simulink model "HEV"  (R2015a)
settings: Solver=ode23tb  StartTime=0.0  StopTime=318  FixedStep=Ts  MaxStep=Ts  RelTol=1  AbsTol=0.5
InitFcn:
  | Ts = 6e-05;   % time step
  | DriveCycleNumber = 1;
  | beginningSim = 1;
undefined symbols (not defined in the file): drive_block, drive_enginemodel, EngineSpeedPower, FuelConsTable, GasEmisTable, h, Hydride, km, magnitude, Metal, Nickel, rad, s, speed, torque
libraries: powerlib x47, driveline x30, simulink x13, simulink_extras x9, electricdrivelib x3, powerlib_extras x3, aerolibconvert2 x2, DC6DriveInternalModels x1
(part 3 of 3)

== system HEV/Electric Motor Controller /Motor 50kW/Three-phase Inverter/Activation Switches ==
  gate : Inport
  Ideal Switch1 : powerlib/Power Electronics/Ideal Switch  Ron=2*Ron  Lon=0  IC=1  Rs=1e6  Cs=inf  Measurements=off
  Ideal Switch2 : powerlib/Power Electronics/Ideal Switch  Ron=2*Ron  Lon=0  IC=1  Rs=1e6  Cs=inf  Measurements=off
  Ideal Switch3 : powerlib/Power Electronics/Ideal Switch  Ron=2*Ron  Lon=0  IC=1  Rs=1e6  Cs=inf  Measurements=off
  Ideal Switch4 : powerlib/Power Electronics/Ideal Switch  Ron=2*Ron  Lon=0  IC=0  Rs=1e6  Cs=inf  Measurements=off
  Ideal Switch5 : powerlib/Power Electronics/Ideal Switch  Ron=2*Ron  Lon=0  IC=0  Rs=1e6  Cs=inf  Measurements=off
  Ideal Switch6 : powerlib/Power Electronics/Ideal Switch  Ron=2*Ron  Lon=0  IC=0  Rs=1e6  Cs=inf  Measurements=off
  Logical Operator : Logic  Operator=NOT  AllPortsSameDT=off  OutDataTypeStr=boolean
  A1 : PMIOPort  Port=1  Side=Left
  a : PMIOPort  Port=2  Side=Right
  B1 : PMIOPort  Port=3  Side=Left
  b : PMIOPort  Port=4  Side=Right
  C1 : PMIOPort  Port=5  Side=Left
  c : PMIOPort  Port=6  Side=Right
  A2 : PMIOPort  Port=7  Side=Left
  B2 : PMIOPort  Port=8  Side=Left
  C2 : PMIOPort  Port=9  Side=Left
  wires:
  gate/1 -> Ideal Switch1/1, Ideal Switch2/1, Ideal Switch3/1, Logical Operator/1
  Logical Operator/1 -> Ideal Switch4/1, Ideal Switch5/1, Ideal Switch6/1
  connections:
  A1/RConn1 -- Ideal Switch1/LConn1
  Ideal Switch1/RConn1 -- a/RConn1 -- Ideal Switch4/RConn1
  B1/RConn1 -- Ideal Switch2/LConn1
  Ideal Switch2/RConn1 -- Ideal Switch5/RConn1 -- b/RConn1
  C1/RConn1 -- Ideal Switch3/LConn1
  Ideal Switch3/RConn1 -- Ideal Switch6/RConn1 -- c/RConn1
  A2/RConn1 -- Ideal Switch4/LConn1
  B2/RConn1 -- Ideal Switch5/LConn1
  C2/RConn1 -- Ideal Switch6/LConn1

== system HEV/Electric Motor Controller /Motor 50kW/Three-phase Inverter/Id computation ==
  m : Inport
  Vdc : Inport  Port=2
  Demux : Subsystem
  Demux1 : Subsystem
  Gain : Gain  Gain=Ron
  Math Function : Math  Operator=magnitude^2  SaturateOnIntegerOverflow=on
  Math Function1 : Math  Operator=magnitude^2  SaturateOnIntegerOverflow=on
  Math Function2 : Math  Operator=magnitude^2  SaturateOnIntegerOverflow=on
  Product1 : Product  Inputs=*/  SaturateOnIntegerOverflow=on  OutDataTypeStr=Inherit: Same as first input
  Sum1 : Sum  Inputs=+++  SaturateOnIntegerOverflow=on
  Sum2 : Sum  Inputs=|++  SaturateOnIntegerOverflow=on
  Sum3 : Sum  SaturateOnIntegerOverflow=on
  Unit Delay1 : UnitDelay  SampleTime=Ts
  Unit Delay4 : UnitDelay  InitialCondition=1  SampleTime=Ts
  Vac x Ia : Product  SaturateOnIntegerOverflow=on  OutDataTypeStr=Inherit: Same as first input
  Vbc x Ib : Product  SaturateOnIntegerOverflow=on  OutDataTypeStr=Inherit: Same as first input
  Zero avoider : Saturate  UpperLimit=inf  LowerLimit=1
  Id : Outport
  wires:
  Sum2/1 -> Unit Delay1/1
  Sum3/1 -> Sum2/1
  Sum1/1 -> Gain/1
  Math Function2/1 -> Sum1/3
  Math Function/1 -> Sum1/1
  Math Function1/1 -> Sum1/2
  Demux1/3(Ic) -> Math Function2/1
  Demux1/2(Ib) -> Math Function1/1
  Demux1/1(Ia) -> Math Function/1
  Unit Delay4/1 -> Zero avoider/1
  Unit Delay1/1 -> Product1/1
  m/1 -> Demux1/1(m), Demux/1(m)
  Vac x Ia/1 -> Sum3/1
  Vbc x Ib/1 -> Sum3/2
  Vdc/1 -> Unit Delay4/1
  Demux/1(Vac) -> Vac x Ia/1
  Demux/2(Ia) -> Vac x Ia/2
  Demux/4(Ib) -> Vbc x Ib/2
  Demux/3(Vbc) -> Vbc x Ib/1
  Gain/1 -> Sum2/2
  Product1/1 -> Id/1
  Zero avoider/1 -> Product1/2

== system HEV/Electric Motor Controller /Motor 50kW/Three-phase Inverter/Limit detection ==
  note: Limit = 1 saturation mode (voltage mode)
      | Limit = 0 normal mode (current mode)
  note: Low pass filter
  note: Low pass filter
  Vcc : Inport
  ctrl : Inport  Port=2
  Bus Selector1 : BusSelector  OutputSignals=m.Stator current is_d (A),m.Stator current is_q (A),m.Rotor speed wm (rad/s)  OutputAsBus=on
  Discrete Transfer Fcn1 : DiscreteTransferFcn  Numerator=[1-exp(-Ts*Fcs*2*pi)]  Denominator=[1 -exp(-Ts*Fcs*2*pi)]  SampleTime=Ts
  Discrete Transfer Fcn3 : DiscreteTransferFcn  Numerator=[1-exp(-Ts*Fcs*2*pi)]  Denominator=[1 -exp(-Ts*Fcs*2*pi)]  SampleTime=Ts
  Gain1 : Gain  Gain=0.9  SaturateOnIntegerOverflow=on  OutDataTypeStr=Inherit: Same as input  ParamDataTypeStr=Inherit: Same as input
  "Internal Vcc " : Fcn  Expr=pi/2*sqrt((Resistance*u(1)-Lq*p*u(3)*u(2))^2+(Resistance*u(2)+Ld*p*u(3)*u(1)+Flux*p*u(3))^2)
  Relational Operator : RelationalOperator  Operator=>  OutDataTypeStr=boolean
  Relational Operator2 : RelationalOperator  Operator=<  OutDataTypeStr=boolean
  S-R Flip-Flop : simulink_extras/Flip Flops/S-R Flip-Flop  initial_condition=0
  Terminator : Terminator
  Limit : Outport
  wires:
  Vcc/1 -> Discrete Transfer Fcn3/1
  Relational Operator/1 -> S-R Flip-Flop/1
  Relational Operator2/1 -> S-R Flip-Flop/2
  S-R Flip-Flop/1 -> Limit/1
  ctrl/1 -> Bus Selector1/1
  Bus Selector1/1 -> "Internal Vcc "/1
  "Internal Vcc "/1 -> Discrete Transfer Fcn1/1
  Discrete Transfer Fcn1/1 -> Relational Operator/1, Relational Operator2/1
  Gain1/1 -> Relational Operator2/2
  Discrete Transfer Fcn3/1 -> Gain1/1, Relational Operator/2
  S-R Flip-Flop/2 -> Terminator/1

== system HEV/Electric Motor Controller /Motor 50kW/Three-phase Inverter/Output Resistance correction ==
  note: Vabc
  ctrl : Inport
  1/R : Gain  Gain=1/(100*Resistance)  SaturateOnIntegerOverflow=on  OutDataTypeStr=Inherit: Same as input  ParamDataTypeStr=Inherit: Same as input
  Bus Selector1 : BusSelector  OutputSignals=m.Stator voltage Vs_d (V),m.Stator voltage Vs_q (V),m.Rotor angle thetam (rad)
  Constant : Constant  Value=0
  Discrete Transfer Fcn1 : DiscreteTransferFcn  Numerator=[1-exp(-Ts/.001)]  Denominator=[1 -exp(-Ts/.001)]  SampleTime=Ts
  Discrete Transfer Fcn2 : DiscreteTransferFcn  Numerator=[1-exp(-Ts/.001)]  Denominator=[1 -exp(-Ts/.001)]  SampleTime=Ts
  Fcn : Fcn  Expr=sin(u)
  Fcn1 : Fcn  Expr=cos(u)
  Mux4 : Mux  Inputs=3
  Mux5 : Mux  Inputs=2
  dq0_to_abc Transformation : powerlib_extras/Measurements/dq0_to_abc Transformation
  poles : Gain  Gain=p  SaturateOnIntegerOverflow=on  OutDataTypeStr=Inherit: Same as input  ParamDataTypeStr=Inherit: Same as input
  "Iabc_r " : Outport
  wires:
  1/R/1 -> "Iabc_r "/1
  Bus Selector1/2 -> Discrete Transfer Fcn2/1  "<Stator voltage Vs_q (V)>"
  Bus Selector1/1 -> Discrete Transfer Fcn1/1  "<Stator voltage Vs_d (V)>"
  ctrl/1 -> Bus Selector1/1
  Mux4/1 -> dq0_to_abc Transformation/1
  Fcn/1 -> Mux5/1
  Fcn1/1 -> Mux5/2
  Mux5/1 -> dq0_to_abc Transformation/2
  Constant/1 -> Mux4/3
  dq0_to_abc Transformation/1 -> 1/R/1
  Discrete Transfer Fcn2/1 -> Mux4/2
  Discrete Transfer Fcn1/1 -> Mux4/1
  Bus Selector1/3 -> poles/1  "<Rotor angle thetam (rad)>"
  poles/1 -> Fcn1/1, Fcn/1

== system HEV/Electric Motor Controller /Motor 50kW/VECT controller/Current Regulator ==
  Iabc* : Inport
  Iabc : Inport  Port=2
  Demux1 : Demux  Outputs=3
  Demux2 : Demux  Outputs=3
  Mux1 : Mux  Inputs=2
  Relay : Relay  OnSwitchValue=0  OffSwitchValue=0
  Relay1 : Relay  OnSwitchValue=0  OffSwitchValue=0
  Relay2 : Relay  OnSwitchValue=0  OffSwitchValue=0
  Sum : Sum  Inputs=-+  SaturateOnIntegerOverflow=on  InputSameDT=on  OutDataTypeStr=Inherit: Same as first input
  Sum1 : Sum  Inputs=-+  SaturateOnIntegerOverflow=on  InputSameDT=on  OutDataTypeStr=Inherit: Same as first input
  Sum2 : Sum  Inputs=-+  SaturateOnIntegerOverflow=on  InputSameDT=on  OutDataTypeStr=Inherit: Same as first input
  Sum3 : Sum  Inputs=+-
  Sum4 : Sum  Inputs=+-
  Pulses : Outport  InitialOutput=0
  wires:
  Sum/1 -> Relay/1
  Sum1/1 -> Relay1/1
  Demux1/1 -> Sum/1
  Demux1/2 -> Sum1/1
  Mux1/1 -> Pulses/1
  Iabc/1 -> Demux1/1
  Sum2/1 -> Relay2/1
  Demux1/3 -> Sum2/1
  Demux2/3 -> Sum2/2
  Demux2/2 -> Sum1/2
  Demux2/1 -> Sum/2
  Iabc*/1 -> Demux2/1
  Relay/1 -> Sum3/1
  Relay1/1 -> Sum3/2, Sum4/1
  Relay2/1 -> Sum4/2
  Sum3/1 -> Mux1/1
  Sum4/1 -> Mux1/2

== system HEV/Electric Motor Controller /Motor 50kW/VECT controller/DQ-ABC ==
  "Iq* " : Inport
  "Id* " : Inport  Port=2
  Teta : Inport  Port=3
  Fcn : Fcn  Expr=sin(u)
  Fcn1 : Fcn  Expr=cos(u)
  Gain2 : Gain  SaturateOnIntegerOverflow=on  OutDataTypeStr=Inherit: Same as input  ParamDataTypeStr=Inherit: Same as input
  Gain3 : Gain  SaturateOnIntegerOverflow=on  OutDataTypeStr=Inherit: Same as input  ParamDataTypeStr=Inherit: Same as input
  Gain4 : Gain  SaturateOnIntegerOverflow=on  OutDataTypeStr=Inherit: Same as input  ParamDataTypeStr=Inherit: Same as input
  Mux : Mux
  Mux2 : Mux  Inputs=3
  ia : Fcn  Expr=-u[3]*u[2] + u[4]*u[1]
  ib : Fcn  Expr=(-u[1]+1.7320508*u[2])*u[4]*0.5+(u[2]+1.7320508*u[1])*u[3]*0.5
  ic : Sum  Inputs=--  SaturateOnIntegerOverflow=on  InputSameDT=on  OutDataTypeStr=Inherit: Same as first input
  Iabc* : Outport  InitialOutput=0
  wires:
  Fcn/1 -> Mux/2
  Fcn1/1 -> Mux/1
  Mux2/1 -> Iabc*/1
  Mux/1 -> ib/1, ia/1
  Teta/1 -> Fcn1/1, Fcn/1
  "Id* "/1 -> Mux/3
  "Iq* "/1 -> Mux/4
  Gain3/1 -> Mux2/2
  ic/1 -> Gain4/1
  Gain4/1 -> Mux2/3
  Gain2/1 -> Mux2/1
  ia/1 -> Gain2/1, ic/2
  ib/1 -> Gain3/1, ic/1

== system HEV/Electric Motor Controller /Motor 50kW/VECT controller/Zero crossing detector ==
  En : Inport
  Iabc* : Inport  Port=2
  D Latch : simulink_extras/Flip Flops/D Latch
  D Latch1 : simulink_extras/Flip Flops/D Latch
  D Latch2 : simulink_extras/Flip Flops/D Latch
  Data Type Conversion : DataTypeConversion
  Data Type Conversion2 : DataTypeConversion
  Demux : Demux  Outputs=3
  Hit Crossing : HitCross
  Mux : Mux  Inputs=3
  Terminator : Terminator
  Terminator1 : Terminator
  Terminator2 : Terminator
  Enable : Outport
  wires:
  Data Type Conversion/1 -> D Latch/1, D Latch1/1, D Latch2/1
  Hit Crossing/1 -> Demux/1
  Demux/2 -> D Latch1/2
  Demux/3 -> D Latch2/2
  D Latch/1 -> Mux/1
  D Latch1/1 -> Mux/2
  D Latch2/1 -> Mux/3
  Mux/1 -> Data Type Conversion2/1
  Demux/1 -> D Latch/2
  En/1 -> Data Type Conversion/1
  Iabc*/1 -> Hit Crossing/1
  Data Type Conversion2/1 -> Enable/1
  D Latch/2 -> Terminator/1
  D Latch1/2 -> Terminator1/1
  D Latch2/2 -> Terminator2/1

== system HEV/Electric Motor Controller /Generator 30kW/Three-phase Inverter/Id computation/Demux ==
  m : Inport
  Demux1 : Demux  Outputs=5
  Terminator : Terminator
  Vac : Outport
  Ia : Outport  Port=2
  Vbc : Outport  Port=3
  Ib : Outport  Port=4
  wires:
  Demux1/3 -> Terminator/1  "Ic"
  Demux1/1 -> Ia/1  "Ia"
  Demux1/2 -> Ib/1  "Ib"
  Demux1/4 -> Vac/1  "Vac"
  Demux1/5 -> Vbc/1  "Vbc"
  m/1 -> Demux1/1

== system HEV/Electric Motor Controller /Generator 30kW/Three-phase Inverter/Id computation/Demux1 ==
  m : Inport
  Demux1 : Demux  Outputs=5
  Terminator1 : Terminator
  Terminator2 : Terminator
  Ia : Outport
  Ib : Outport  Port=2
  Ic : Outport  Port=3
  wires:
  m/1 -> Demux1/1
  Demux1/5 -> Terminator2/1  "Vbc"
  Demux1/4 -> Terminator1/1  "Vac"
  Demux1/2 -> Ib/1  "Ib"
  Demux1/1 -> Ia/1  "Ia"
  Demux1/3 -> Ic/1  "Ic"

== system HEV/Electric Motor Controller /Motor 50kW/Three-phase Inverter/Id computation/Demux ==
  m : Inport
  Demux1 : Demux  Outputs=5
  Terminator : Terminator
  Vac : Outport
  Ia : Outport  Port=2
  Vbc : Outport  Port=3
  Ib : Outport  Port=4
  wires:
  m/1 -> Demux1/1
  Demux1/5 -> Vbc/1  "Vbc"
  Demux1/4 -> Vac/1  "Vac"
  Demux1/2 -> Ib/1  "Ib"
  Demux1/1 -> Ia/1  "Ia"
  Demux1/3 -> Terminator/1  "Ic"

== system HEV/Electric Motor Controller /Motor 50kW/Three-phase Inverter/Id computation/Demux1 ==
  m : Inport
  Demux1 : Demux  Outputs=5
  Terminator1 : Terminator
  Terminator2 : Terminator
  Ia : Outport
  Ib : Outport  Port=2
  Ic : Outport  Port=3
  wires:
  Demux1/3 -> Ic/1  "Ic"
  Demux1/1 -> Ia/1  "Ia"
  Demux1/2 -> Ib/1  "Ib"
  Demux1/4 -> Terminator1/1  "Vac"
  Demux1/5 -> Terminator2/1  "Vbc"
  m/1 -> Demux1/1

== matlab function HEV/Power Controller/Game Theory Controller/MATLAB Function ==
  data: requiredTorque input double size=[1 1]; SOC input double; fuelConsumed input; engineTorque output; motorTorque output; FuelConsTable parameter; GasEmisTable parameter
function [engineTorque,motorTorque] = solveGame(requiredTorque, SOC, fuelConsumed, FuelConsTable, GasEmisTable)
%#codegen
    coder.extrinsic('int2str');
    coder.extrinsic('ismembertol');
    coder.extrinsic('knnsearch'); 
    coder.extrinsic('legend');
    coder.extrinsic('roundn');
    requiredTorqueR = 0;
    requiredTorqueR = roundn(requiredTorque,0);     
        
    %if previousReqTorque == requiredTorqueR
    %    engineTorque = previousEngTorque;
    %    motorTorque = previousMotTorque;
    %else
        if requiredTorqueR > 0 && requiredTorqueR <= 70 
           requiredTorqueR = 70;
           engineTorque = 0;
           motorTorque = requiredTorqueR;
        elseif requiredTorqueR > 70 && requiredTorqueR < 83
           engineTorque = 0;
           motorTorque = requiredTorqueR;
        elseif requiredTorqueR < 0          
           engineTorque = 0;
           motorTorque = requiredTorqueR;
        elseif requiredTorqueR == 0          
            engineTorque = 0;
            motorTorque = 0;
        else
            close all   
            motorSpeedCurve = [0, 1200, 2000, 3000, 4000, 5000, 6000];
            motorTorqueCurve = [400 399 225 150 100 80 70];

            SOC_deviation = abs(70 - SOC);       
            maxEngineTorque = 136;
            maxMotorTorque = 400;
            minMotorTorque = -400;
            minMotorTorqueRef = 0;
            minEngineTorqueRef = 83;
            minEngineTorque = 83;
            m = 7;
            e = 7;
            payoffMotor = zeros(m,e);
            payoffEngine = zeros(m,e);      
            if requiredTorque < 0
                maxMotorTorqueStrategy = 0;
                maxEngineTorqueStrategy = 0;
                minEngineTorqueStrategy = max(minEngineTorque, requiredTorque); 
                minMotorTorqueStrategy = max(minMotorTorque, requiredTorque);  
                strategyMot = linspace(minMotorTorqueStrategy, maxMotorTorqueStrategy, m);
                strategyEng = linspace(minEngineTorqueStrategy, maxEngineTorqueStrategy,e);
            else
                minEngineTorqueStrategy = 0;
                minMotorTorqueStrategy = 0;
                maxEngineTorqueStrategy = min([requiredTorque maxEngineTorque]);
                maxMotorTorqueStrategy = min([requiredTorque maxMotorTorque]);    
                if minMotorTorqueRef > maxMotorTorqueStrategy
                    strategyMot = zeros(1,m);
                else
                    strategyMot = linspace(minMotorTorqueRef, maxMotorTorqueStrategy, m);
                end
                if minEngineTorqueRef > maxEngineTorqueStrategy
                    strategyEng = zeros(1,e);
                else
                    strategyEng = linspace(minEngineTorqueRef, maxEngineTorqueStrategy,e);
                end
            end          
            
            tmpTorque = repmat(strategyEng',1,m);

            totalTorque = zeros(m, e);
            for i = 1:m
                for j = 1:e
                    totalTorque(i,j) = tmpTorque(i,j) + strategyMot(j);
                end
            end      

            % weights     
            wFuel = 3;
            wPower = 0.5;  
            wTank = 0.5;
            wDrDem = 0.5;
            wSOC = 1;
            wNOX = 65;
            wCO = 25;
            wHC = 45;
            motorSpeedRef = zeros(1,e);
            powerMotorKW = zeros(1,e);
            torqueDeviation = zeros(m,e);
            fuel = zeros(e,1);
            nox = zeros(e,1);
            power = zeros(e,1);

            for i = 1:m
                for j = 1:e
                    tmpT = abs(FuelConsTable.torque - strategyEng(j));
                    idxT = 0;                    
                    % Power(W) = Torque (N.m) x Speed (RPM) / 9.5488
                    % divide by 1000 for kW               
                    motorSpeedRef(j) = interp1(motorTorqueCurve, motorSpeedCurve, abs(strategyMot(j)),'linear','extrap');
                    powerMotorKW(j) = abs(strategyMot(j)) * motorSpeedRef(j) / 9.5488 / 1000;       
                    tmpS = abs(FuelConsTable.speed - motorSpeedRef(j));
                    idxS = 0;
                    [~, idxS] = min(tmpS);
                    [~, idxT] = min(tmpT);    

                    fuelConsumedGPS = FuelConsTable.lookupTableFuel(idxT, idxS);
                    HCEmissions = GasEmisTable.lookupTableHC(idxT, idxS);
                    COEmissions = GasEmisTable.lookupTableCO(idxT, idxS);
                    NOXEmissions = GasEmisTable.lookupTableNOX(idxT, idxS);   
                    torqueDeviation(i,j) = requiredTorqueR - totalTorque(i,j);             

                    payoffEngine(i,j) = wFuel*fuelConsumedGPS + wDrDem*abs(torqueDeviation(i,j)) + ...
                        wHC*HCEmissions + wCO*COEmissions + wNOX*NOXEmissions + ...
                        wTank*fuelConsumed;
                    payoffMotor(i,j) = wDrDem*abs(torqueDeviation(i,j)) + wPower*powerMotorKW(j) + ...
                        wSOC*SOC_deviation;              
                    fuel(j,1) = fuelConsumedGPS;
                    nox(j,1) = NOXEmissions;
                    power(j,1) = powerMotorKW(j);                                
                end
            end

            paretoStrategies = [];
            paretoIndex = [];
            payoffEngine;
            payoffMotor;
            [paretoStrategies, paretoIndex, ~, ~] = paretoset(payoffEngine, payoffMotor);       

            payoffE = reshape(payoffEngine,(m)*(e),1);
            payoffM = reshape(payoffMotor,(m)*(e),1);        
            payoffBoth = horzcat(payoffE, payoffM);   

            engineTorquePareto = strategyEng(paretoIndex(:,1));
            motorTorquePareto = strategyMot(paretoIndex(:,2));        
            stringRequiredTorque = int2str(requiredTorqueR);   

            [ bestPayoffEngPareto, bestPayoffMotPareto ] = bestpareto( paretoStrategies, paretoIndex, ...
            torqueDeviation, fuel, nox, power );


    %         numStratBoth = m+e;  
    %        
    %         [nashEqPl1, nashEqPl2] = LemkeHowson(-payoffEngine, -payoffMotor, ceil(1/2*numStratBoth));                     
    %         payoffEngNash = payoffEngine(nashEqPl1==1, nashEqPl2==1);
    %         payoffMotNash = payoffMotor(nashEqPl1==1, nashEqPl2==1);       
    %         %[~, indM] = min(payoffEngNash);        
    %               
    %         conflictPoint = sub2ind([m e], find(nashEqPl1==1), find(nashEqPl2==1));
    %         
    %         [~, indNP] = nashsolution(payoffBoth, conflictPoint);
    %         payoffEngNashSol = payoffBoth(indNP,1);
    %         payoffMotNashSol = payoffBoth(indNP,2);
    %         paretoStrInd = horzcat(paretoStrategies, paretoIndex);        
    % 
    %         [ks, linePareto] = kalaismorodinskysolution(payoffBoth, conflictPoint, paretoStrategies, paretoStrInd);
    %         percentReqTorq = linspace(0, requiredTorqueR, 10);
    %         probKsMixed = zeros(1,2);
    %         ksMixed = zeros(1,2);
    %         if ~isempty(linePareto)
    %             if linePareto(2,1) - linePareto(1,1) ~=0 && linePareto(1,2) - linePareto(2,2) ~= 0
    %                 probKsMixed(1) = (ks(1,1) - linePareto(1,1)) / (linePareto(2,1) - linePareto(1,1));
    %                 probKsMixed(2) = (ks(1,2) - min(linePareto(:,2))) / (linePareto(1,2) - linePareto(2,2));
    %             elseif linePareto(2,1) - linePareto(1,1) == 0
    %                 probKsMixed(2) = (ks(1,2) - min(linePareto(:,2))) / (linePareto(1,2) - linePareto(2,2));
    %                 probKsMixed(1) = 1 - probKsMixed(2);
    %             elseif linePareto(1,2) - linePareto(2,2) == 0
    %                  probKsMixed(1) = (ks(1,1) - linePareto(1,1)) / (linePareto(2,1) - linePareto(1,1));
    %                  probKsMixed(2) = 1 - probKsMixed(1);
    %             end             
    %             ksMixed(1) = linePareto(1,1) + probKsMixed(1)*(linePareto(2,1) - linePareto(1,1));
    %             ksMixed(2) = min(linePareto(:,2)) + probKsMixed(2)*abs(linePareto(1,2) - linePareto(2,2));
    %                         
    %             mixedEngineTorque = min(strategyEng(linePareto(1,3)),strategyEng(linePareto(2,3))) + ...
    %                 probKsMixed(1)*abs(strategyEng(linePareto(1,3))-strategyEng(linePareto(2,3)));
    %             mixedMotorTorque = min(strategyMot(linePareto(1,4)),strategyMot(linePareto(2,4))) + ...
    %                 probKsMixed(1)*abs(strategyMot(linePareto(1,4))-strategyMot(linePareto(2,4)));
    %         end
    %         
    %         %payoffCoalCoef = ones(m,e);
    %         %payoffCoalCoef(m:m-1:end-1) = 0.5;
    %         
    %         [ payoffWholeCoal, coeffCoal, payoffEngineCoal, payoffMotorCoal, payoffWholeCoalBefore ] = ...
    %             coalitionpayoffs(payoffMotor, payoffEngine, torqueDeviation, percentReqTorq);
    %         
    %         indCoal = (coeffCoal == 0.99 | coeffCoal == 0.991);
    %         indCoalition = +indCoal;
    %         indCoalition(indCoal == true) = 0.98;
    %         indCoalition(indCoal == false) = 1;
    %         %payoffWholeCoal1 = payoffWholeCoal .* indCoalition;      
    %     
    %         payoffMotCoalVec = reshape(payoffMotorCoal,(m)*(e),1);
    %         payoffEngCoalVec = reshape(payoffEngineCoal,(m)*(e),1);
    %         
    %         % get all undominated strategies (pareto optimality)
    %         [undomImp, undomImpInd] = checkimputation(payoffBoth, ...
    %             paretoStrategies, payoffMotCoalVec, payoffEngCoalVec, payoffWholeCoal);        
    %         imputM = zeros(1,size(undomImpInd,2));
    %         imputE = zeros(1,size(undomImpInd,2));
    %         for i = 1 : size(undomImpInd,2)             
    %             if all(undomImp(i,1) <= payoffEngine(m,:))
    %                 imputM(1,i) = undomImpInd(i);
    %             end                
    %             if all(undomImp(i,2) <= payoffMotor(:,e))
    %                 imputE(1,i) = undomImpInd(i);
    %             end
    %         end
    %         coder.varsize('imput');  
    %         imput = undomImpInd;
    %         imput(imput==0) = [];
    %         
    %         payoffImput = zeros(size(imput,1),3);
    %         for i = 1 : size(imput,1)
    %             payoffImput(i,1) = payoffBoth(imput(i),1);
    %             payoffImput(i,2) = payoffBoth(imput(i),2);       
    %             [r, c] = ind2sub(size(payoffWholeCoal), imput(i));
    %             payoffImput(i,3) = payoffWholeCoal(r,c);
    %         end
    %                
    %         coreSol = core(payoffImput);
    %         indCore = find(coreSol);
    %         Xengine = zeros(m,1);
    %         Xmotor = zeros(m,1);
    %         [Xengine, X2, A1, b1, v1] = mixedstrategies(payoffEngine,1);
    %         [Xmotor, X1, A2, b2, v2] = mixedstrategies(payoffMotor,2);
    %         coder.varsize('payoffStrEng');
    %         coder.varsize('payoffStrMot');        
    %        
    %         if  ~isempty(A1) && ~isempty(A2) && ~isempty(b1) && ~isempty(b2)
    %             mixedStrEng = find(abs(Xengine-0)>0.001);
    %             mixedStrMot = find(abs(Xmotor-0)>0.001);         
    %             payoffProbMixedStrEng = zeros(size(mixedStrEng,1),2);
    %             payoffProbMixedStrMot = zeros(size(mixedStrMot,1),2);
    %             payoffStrEng = 0;
    %             for i = 1 : size(mixedStrEng,1)        
    %                 payoffProbMixedStrEng(i,1) = payoffEngine(mixedStrEng(i));
    %                 payoffProbMixedStrEng(i,2) = Xengine(mixedStrEng(i));
    %                 payoffStrEng = payoffStrEng + payoffEngine(mixedStrEng(i))*Xengine(mixedStrEng(i));
    %             end
    % 
    %             payoffStrMot = 0;
    %             for j = 1 : size(mixedStrMot,1)
    %                 payoffProbMixedStrMot(j,1) = payoffMotor(mixedStrMot(j));
    %                 payoffProbMixedStrMot(j,2) = Xmotor(mixedStrMot(j));    
    %                 payoffStrMot = payoffStrMot + payoffMotor(mixedStrMot(j))*Xmotor(mixedStrMot(j));
    %             end         
    %         else
    %             pureStrEng = find(Xengine);
    %             pureStrMot = find(X2);    
    %             payoffStrEng = payoffEngine(pureStrEng, pureStrMot);
    %             payoffStrMot = payoffMotor(pureStrEng, pureStrMot);           
    %         end
    %         m1 = min(payoffBoth(:,1));
    %         m2 = min(payoffBoth(:,2));
    % 
    %         v12 = min(min(payoffWholeCoalBefore));
    %         [ shEngine, shMotor ] = shapleyvalue(v12, v1, v2);
    %         if ~ismembertol([shEngine, shMotor],payoffBoth,0.001,'ByRows',true)           
    %             IDX = zeros(1,2);
    %             IDX = knnsearch(payoffBoth,[shEngine shMotor],'K', 2);
    %             [idr1, idc1] = ind2sub(size(payoffEngine), IDX(1));        
    %             [idr2, idc2] = ind2sub(size(payoffEngine), IDX(2));
    %             nearestSh1 = [idr1 idc1];
    %             nearestSh2 = [idr2 idc2];
    %             payoffNearestSh1 = [payoffEngine(idr1,idc1) payoffMotor(idr1,idc1)];
    %             payoffNearestSh2 = [payoffEngine(idr2,idc2) payoffMotor(idr2,idc2)];
    %             probNearSh1 = 0;
    %             probNearSh2 = 0;
    %             if payoffNearestSh1(1) ~= payoffNearestSh2(1)
    %                 j = 1;
    %                 shapley = shEngine;
    %             else
    %                 j = 2;
    %                 shapley = shMotor;
    %             end
    %             if payoffNearestSh2(j) < shapley &&  ...
    %                 shapley < payoffNearestSh1(j)
    %                 probNearSh2 = (shapley - payoffNearestSh2(j)) / ...
    %                     (payoffNearestSh1(j) - payoffNearestSh2(j));
    %                 probNearSh1 = 1 - probNearSh2;
    %             elseif payoffNearestSh1(j) < shapley && ...                    
    %                 shapley < payoffNearestSh2(j)
    %                 probNearSh1 = (shapley - payoffNearestSh1(j)) / ...
    %                     (payoffNearestSh2(j) - payoffNearestSh1(j));
    %                 probNearSh2 = 1 - probNearSh1;
    %             elseif shapley < payoffNearestSh1(j) &&  ...
    %                 shapley < payoffNearestSh2(j)            
    %                 if payoffNearestSh1(j) < payoffNearestSh2(j)
    %                     probNearSh1 = shapley / payoffNearestSh1(j);
    %                     probNearSh2 = 0;
    %                 elseif payoffNearestSh2(j) < payoffNearestSh1(j)
    %                     probNearSh2 = shapley / payoffNearestSh2(j);
    %                     probNearSh1 = 0;
    %                 end
    %             end
    %             probNearSh1;
    %             probNearSh2;
    %             shapleyEngineTorque = probNearSh1*strategyEng(idr1) + probNearSh2*strategyEng(idr2);
    %             shapleyMotorTorque = probNearSh1*strategyMot(idc1) + probNearSh2*strategyMot(idc2);          
    %         else
    %              [~, ind] = ismembertol([shEngine, shMotor],payoffBoth,0.001,'ByRows',true); 
    %              idr1 = 0;
    %              idc1 = 0;
    %              [idr1, idc1] = ind2sub(size(payoffEngine), ind);             
    %              shapleyEngineTorque = strategyEng(idr1);
    %              shapleyMotorTorque = strategyMot(idc1);    
    %         end

            %lightpurple = [163 154 255] ./ 255;        
            %p10 = plot(payoffStrEng, payoffStrMot, 'o',...
            %    'MarkerFaceColor', lightpurple, 'MarkerEdgeColor', lightpurple, ...
            %    'MarkerSize', 13);

            %limegreen = [194 242 1] ./ 255;
            %p3 = plot(bestPayoffEngPareto, bestPayoffMotPareto, 'og', ...
            %    'MarkerFaceColor', 'g', 'MarkerSize', 12);    
            %p5 = plot(payoffEngNashNPG, payoffMotNashNPG, 'o', ...
            %    'MarkerFaceColor','m', 'MarkerEdgeColor', 'm',...
            %    'MarkerSize', 13);    
            %p4 = plot(payoffEngNash, payoffMotNash, 'oy', ...
            %    'MarkerFaceColor', 'y', 'MarkerSize', 10);     
            %p41 = plot(bestPayoffEngNashLH(1), bestPayoffMotNashLH(1), 'oc', ...
            %    'MarkerFaceColor', 'c', 'MarkerSize', 9);      
            %p42 = plot(bestPayoffEngNashLH(2), bestPayoffMotNashLH(2), 'o', ...
            %    'MarkerFaceColor', 'r', 'MarkerEdgeColor','r','MarkerSize', 7);     
            %p43 = plot(bestPayoffEngNashLH(3), bestPayoffMotNashLH(3), 'o', ...
            %    'MarkerFaceColor', limegreen,'MarkerEdgeColor', limegreen, 'MarkerSize', 5);         
            %p6 = plot(payoffEngNashSol, payoffMotNashSol,'or', ...
            %    'MarkerFaceColor',[1,0.6,0] , 'MarkerEdgeColor', [1,0.6,0] ,...
            %    'MarkerSize', 9);

            %purple = [118 31 133] ./ 255;        
            %p7 = plot(ks(1,1), ks(1,2), 'o', 'MarkerFaceColor', purple, ...
            %    'MarkerEdgeColor', purple, 'MarkerSize', 9);
            %pink = [254 164 191] ./ 255;       
            %p8 = plot(payoffBoth(imput(indCore),1), payoffBoth(imput(indCore),2), 'o', ...
            %    'MarkerFaceColor',pink, 'MarkerEdgeColor',pink,...
            %    'MarkerSize', 8);      

            %p9 = plot(shEngine, shMotor, 'o', 'MarkerFaceColor', limegreen, ...
            %    'MarkerEdgeColor', limegreen, 'MarkerSize', 7);
            %p2 = p9;

            %for r = 1 : size(paretoIndex,1)
            %    linearIndex = sub2ind([m e], paretoIndex(r,2), paretoIndex(r,1));           
            %    p2 = plot(x(linearIndex), y(linearIndex), 'o', ...
            %        'MarkerEdgeColor', [0,0.5,0], 'MarkerFaceColor',[0,0.5,0],...
            %        'MarkerSize',6);
            %end

            %darkred = [185 16 20] ./ 255;
            %pi = plot(m1, m2, 'o', 'MarkerSize', 4, 'MarkerFaceColor',darkred ,...
            %'MarkerEdgeColor', darkred);


            %legend([p1 p2 p3 p4 p7 p8 p9 p10], 'Payoff', ...         
            %'Pareto optimal payoff', ...  
            %'Best Pareto payoff', ... 
            %'Nash Equilibrium Lemke-Howson (conflict point)', ... 
            %'Kalai-Smorodinsky Solution', ...
            %'Core', ...        
            %'Shapley value', ...
            %'Mixed Strategies', ...
            %'Location', 'northwest');       

            %'Ideal point', ...       
            %'Nash Equilibrium Lemke-Howson k0=1', ...
            %'Nash Equilibrium Lemke-Howson k0=8', ...     
            %'Nash Equilibrium Lemke-Howson k0=15' , ... 
            %'Nash Equilibrium Lemke-Howson k0=23' , ...          
            %'Nash Equilibrium NPG', ...       

            %xlabel('Payoff Engine');
            %ylabel('Payoff Motor');
            %hold off
       
            [ engineTorque, motorTorque ] = payofftotorque(bestPayoffEngPareto, ...
                bestPayoffMotPareto, payoffBoth, strategyEng, strategyMot);
            %previousReqTorque = requiredTorqueR;
            %previousEngTorque = engineTorque;
            %previousMotTorque = motorTorque;
       
            %end
        end
    end

== matlab function HEV/Electric Motor Controller /Motor 50kW/VECT controller/MTPA Field Weakening Controller ==
  data: iqn_opt input; Ten input; iqn output; w input; Vdc input; params input; idn output
function [iqn,idn] = fcn(iqn_opt,Ten,w,Vdc,params)
% Maximum Torque Per Ampere (MTPA) Field Weakening Controller

kFact = 0.9;
Ld = params(1);
Lq = params(2);
lam = params(3);
p = params(4);
ib = params(5);
Vs = Vdc/(pi/2)*kFact;
ten = abs(Ten);
iqn = sign(Ten)*iqn_opt;
if Ten == 0 && w == 0
    idn = 0;
elseif iqn == 0
    idn = -(lam*p*w-Vs*kFact)/(p*Ld*w*ib);
else
    idn = 1-Ten/iqn;
end
if sqrt((-Lq*p*w*iqn*ib)^2+(Ld*p*w*idn*ib+lam*p*w)^2) >= Vs 
    vs = Vs;
    k1 = 2*lam*Ld/(ib*Lq^2);
    k2 = Ld^2/Lq^2;
    k3 = lam^2/(ib^2*Lq^2)+k2;
    
    g2 = -vs^2/(p^2*ib^2*Lq^2*w^2) + k1 + k3;
    g3 = -k1*ten-2*ten*k2;
    g4 = k2*ten^2;
    
    a1 = abs(-768*g4^3+384*g4^2*g2^2-48*g4*g2^4-432*g2*g4*g3^2+81*g3^4+12*g3^2*g2^3)^(1/2);
    a2 = (-288*g2*g4+108*g3^2+8*g2^3+12*a1)^(1/3);
    a3 = (-4*g2+a2+48/a2*g4+4/a2*g2^2)^(1/2);
    iqn = (1/12*6^(1/2)*a3+1/12*abs(-48*g2-6*a2-288/a2*g4-24/a2*g2^2-72/a3*g3*6^(1/2))^(1/2));
    iqn = sign(Ten)*iqn;

    idn = 1-Ten/iqn;
end
